simulink model "vanderpol"  (R2020b)
settings: Solver=ode1  StartTime=0.0  StopTime=400  FixedStep=0.002  RelTol=1e-3
values from neighbouring files (symbols this model uses):
  cycleGain = 0.5    [advanced_model_setup.m]    (also in setup_physical.m = 1; simulate_hover.m = 0.2)
libraries: simulink_extras x2
settings Model: Creator=Jacob  LastModifiedBy=256444
settings DataIOCC: ReturnWorkspaceOutputs=off
settings DebuggingCC: UnconnectedInputMsg=none  UnconnectedOutputMsg=none  UnconnectedLineMsg=none
settings ModelReferenceCC: EnableRefExpFcnMdlSchedulingChecks=off

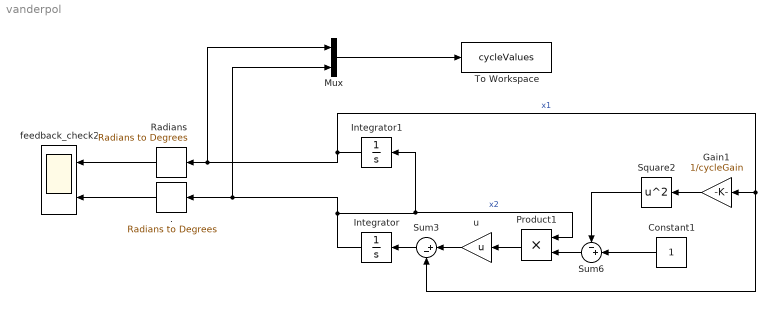
== system vanderpol ==
  . : simulink_extras/Transformations/Radians to Degrees
  Constant1 : Constant
  Gain1 : Gain  Gain=1/cycleGain
  Integrator : Integrator  InitialCondition=0.1
  Integrator1 : Integrator  InitialCondition=0.1
  Mux : Mux  Inputs=2
  Product1 : Product
  Radians : simulink_extras/Transformations/Radians to Degrees
  Square2 : Math  Operator=square  SaturateOnIntegerOverflow=on
  Sum3 : Sum  Inputs=|+-
  Sum6 : Sum  Inputs=-+|
  To Workspace : ToWorkspace  VariableName=cycleValues  SampleTime=-1
  feedback_check2 : Scope  NumInputPorts=2
  u : Gain  Gain=u
  wires:
  Integrator1/1 -> Mux/1, Radians/1, Sum3/2, Gain1/1  "x1"
  Integrator/1 -> Mux/2, ./1, Product1/1, Integrator1/1  "x2"
  Sum3/1 -> Integrator/1
  Sum6/1 -> Product1/2
  Product1/1 -> u/1
  u/1 -> Sum3/1
  Square2/1 -> Sum6/1
  Constant1/1 -> Sum6/2
  ./1 -> feedback_check2/2
  Radians/1 -> feedback_check2/1
  Gain1/1 -> Square2/1
  Mux/1 -> To Workspace/1
